simulink model "KalmanFilter"  (R2019a)
settings: Solver=VariableStepAuto  StartTime=0.0  StopTime=5  RelTol=1e-3
values from neighbouring files (symbols this model uses):
  A = [0 2*g/3/(r+R);1 0]    [Data.m]
  B = [2/3/m/(r+R);0]    [Data.m]
  C = [0 1]    [Data.m]
  D = 0    [Data.m]
  g = 9.81    [Data.m]    (also in func.m; myTransitionFcn.m)
  kR = 1e-3    (= 0.001)    [Data.m]
  m = 0.1    [Data.m]    (also in myTransitionFcn.m)
  r = 0.1    [Data.m]    (also in func.m; myTransitionFcn.m)
  R = 1    [Data.m]    (also in func.m; myTransitionFcn.m)
  Ts = 0.001    [Data.m]
undefined symbols (not defined in the file or in its folder): Continuous, Time
libraries: simulink x2, sharedTrackingLibrary x1, ctrlSharedLib x1
settings Model: Creator=Dell  LastModifiedBy=Dell

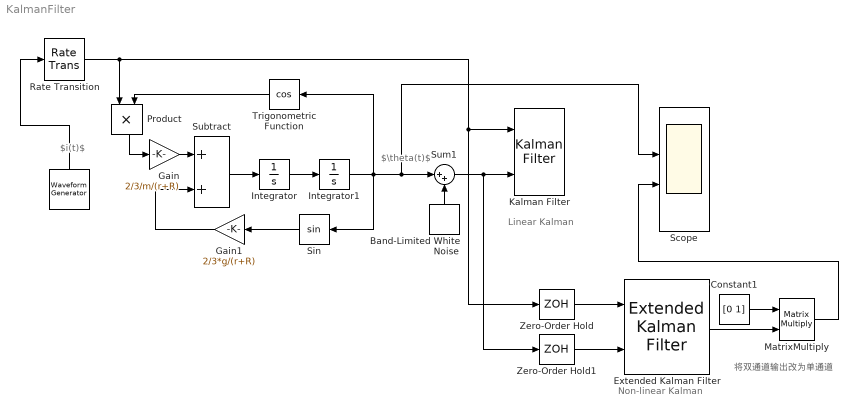
== system KalmanFilter ==
  note: Linear Kalman
  note: 将双通道输出改为单通道
  note: $\theta(t)$
  note: $i(t)$
  note: Non-linear Kalman
  " " : simulink/Sources/Waveform Generator  OutMin=[]  OutMax=[]  OutDataTypeStr=double  SelectedSignal=1  Signals=step(0,0,1)  BlockNames=MultiportSwitch_4fcc108fbbf94f7  SampleTime=Ts
      settings: SourceProductName=Simulink
  Band-Limited White Noise : simulink/Sources/Band-Limited White Noise  Cov=kR  Ts=Ts  seed=[23341]
  Constant1 : Constant  Value=[0 1]  VectorParams1D=off  SampleTime=Ts
  Extended Kalman Filter : sharedTrackingLibrary/Extended Kalman Filter  StateTransitionFcn=myTransitionFcn  HasStateTransitionJacobianFcn=off  HasAdditiveProcessNoise=Additive  ProcessNoise=[0 0]  HasTimeVaryingProcessNoise=off  HasStateTransitionFcnExtraArgument=1  InitialState=[0 0]  InitialStateCovariance=1  MeasurementFcn1=myMeasurementFcn  HasMeasurementJacobianFcn1=off  HasMeasurementEnablePort1=off  HasAdditiveMeasurementNoise1=Additive  MeasurementNoise1=kR  HasTimeVaryingMeasurementNoise1=off  HasMeasurementFcnExtraArgument1=0  MeasurementFcn2=myMeasurementFcn  HasMeasurementJacobianFcn2=off  HasMeasurementEnablePort2=off  HasAdditiveMeasurementNoise2=Additive  MeasurementNoise2=1  HasTimeVaryingMeasurementNoise2=off  HasMeasurementFcnExtraArgument2=0  MeasurementFcn3=myMeasurementFcn  HasMeasurementJacobianFcn3=off  HasMeasurementEnablePort3=off  HasAdditiveMeasurementNoise3=Additive  MeasurementNoise3=1  HasTimeVaryingMeasurementNoise3=off  HasMeasurementFcnExtraArgument3=0  MeasurementFcn4=myMeasurementFcn  HasMeasurementJacobianFcn4=off  HasMeasurementEnablePort4=off  HasAdditiveMeasurementNoise4=Additive  MeasurementNoise4=1  HasTimeVaryingMeasurementNoise4=off  HasMeasurementFcnExtraArgument4=0  MeasurementFcn5=myMeasurementFcn  HasMeasurementJacobianFcn5=off  HasMeasurementEnablePort5=off  HasAdditiveMeasurementNoise5=Additive  MeasurementNoise5=1  HasTimeVaryingMeasurementNoise5=off  HasMeasurementFcnExtraArgument5=0  EnableMultirate=off  StateTransitionFcnSampleTime=1  MeasurementFcn1SampleTime=1  MeasurementFcn2SampleTime=1  MeasurementFcn3SampleTime=1  MeasurementFcn4SampleTime=1  MeasurementFcn5SampleTime=1  UseCurrentEstimator=on  OutputStateCovariance=off  DataType=double  SampleTime=Ts  NumberOfMeasurements=1
      settings: SourceProductName=Control System Toolbox  SourceProductBaseCode=CT
  Gain : Gain  Gain=2/3/m/(r+R)
  Gain1 : Gain  Gain=2/3*g/(r+R)
  Integrator : Integrator
  Integrator1 : Integrator
  Kalman Filter : ctrlSharedLib/Kalman Filter  TimeDomain=Continuous-Time  UseCurrentEstimator=on  ModelSource=Individual A, B, C, D matrices  ModelSourceVariable=ss(0.95,1,1,0,1)  A=A  B=B  C=C  D=D  NumberOfStates=1  NumberOfInputs=1  NumberOfOutputs=1  InitialEstimateSource=Dialog  X0=0  P0=10  UseK=off  UseGH=off  NumberOfProcessNoiseInputs=1  G=1  TimeInvariantG=on  H=0  TimeInvariantH=on  Q=diag([0 0])  TimeInvariantQ=on  R=kR  TimeInvariantR=on  N=0  TimeInvariantN=on  AddInputPort=on  AddEnablePort=off  OutputEstimatedY=off  OutputP=off  Ts=-1
      settings: SourceProductBaseCode=CT
  MatrixMultiply : Product  Multiplication=Matrix(*)
  Product : Product
  Rate Transition : RateTransition
  Scope : Scope  NumInputPorts=4
  Sin : Trigonometry
  Subtract : Sum
  Sum1 : Sum  Inputs=|++
  Trigonometric Function : Trigonometry  Operator=cos
  Zero-Order Hold : ZeroOrderHold  SampleTime=Ts
  Zero-Order Hold1 : ZeroOrderHold  SampleTime=Ts
  wires:
  Gain1/1 -> Subtract/2
  Subtract/1 -> Integrator/1
  Integrator/1 -> Integrator1/1
  Band-Limited White Noise/1 -> Sum1/2
  Sum1/1 -> Zero-Order Hold1/1, Kalman Filter/2
  Integrator1/1 -> Sin/1, Sum1/1, Scope/2, Trigonometric Function/1
  Gain/1 -> Subtract/1
  Trigonometric Function/1 -> Product/2
  Product/1 -> Gain/1
  Sin/1 -> Gain1/1
  Zero-Order Hold/1 -> Extended Kalman Filter/1
  Zero-Order Hold1/1 -> Extended Kalman Filter/2
  Rate Transition/1 -> Zero-Order Hold/1, Kalman Filter/1, Product/1
  Constant1/1 -> MatrixMultiply/1
  Extended Kalman Filter/1 -> MatrixMultiply/2
  MatrixMultiply/1 -> Scope/3
  " "/1 -> Rate Transition/1
